simulink model "InitialSystem_9_Bus"  (R2020a)
settings: Solver=FixedStepAuto  StartTime=0.0  StopTime=Tend  MaxStep=5.0E-5  RelTol=1e-3
values from neighbouring files (symbols this model uses):
  B_s46 = b_s46*Cb    (= 9.5071761847e-07)    [Data_CaseStudyI.m]    (also in Data_CaseStudyII.m; Data_InitialSystem.m)
  B_s54 = b_s54*Cb    (= 1.05902722057e-06)    [Data_CaseStudyI.m]    (also in Data_CaseStudyII.m; Data_InitialSystem.m)
  B_s69 = b_s69*Cb    (= 2.15415764185e-06)    [Data_CaseStudyI.m]    (also in Data_CaseStudyII.m; Data_InitialSystem.m)
  B_s75 = b_s75*Cb    (= 1.84126323577e-06)    [Data_CaseStudyI.m]    (also in Data_CaseStudyII.m; Data_InitialSystem.m)
  B_s87 = b_s87*Cb    (= 8.96562817417e-07)    [Data_CaseStudyI.m]    (also in Data_CaseStudyII.m; Data_InitialSystem.m)
  B_s98 = b_s98*Cb    (= 1.25759482443e-06)    [Data_CaseStudyI.m]    (also in Data_CaseStudyII.m; Data_InitialSystem.m)
  fb = 50    [Data_CaseStudyI.m]    (also in Data_CaseStudyII.m; Data_InitialSystem.m)
  HGov_dyn = HGov_delay*H_tr_droop    [Data_CaseStudyI.m]    (also in Data_CaseStudyII.m; Data_InitialSystem.m)
  HTurb_tot = H_water_way    [Data_CaseStudyI.m]    (also in Data_CaseStudyII.m; Data_InitialSystem.m)
  l1_MVHV1 = 0    [Data_CaseStudyI.m]    (also in Data_CaseStudyII.m; Data_InitialSystem.m)
  l1_MVHV2 = 0    [Data_CaseStudyI.m]    (also in Data_CaseStudyII.m; Data_InitialSystem.m)
  l1_MVHV3 = 0    [Data_CaseStudyI.m]    (also in Data_CaseStudyII.m; Data_InitialSystem.m)
  l2_MVHV1 = l_s14    (= 0.0576)    [Data_CaseStudyI.m]    (also in Data_CaseStudyII.m; Data_InitialSystem.m)
  l2_MVHV2 = l_s72    (= 0.0625)    [Data_CaseStudyI.m]    (also in Data_CaseStudyII.m; Data_InitialSystem.m)
  l2_MVHV3 = l_s39    (= 0.0586)    [Data_CaseStudyI.m]    (also in Data_CaseStudyII.m; Data_InitialSystem.m)
  L_s46 = l_s46*Lb    (= 0.154915055408)    [Data_CaseStudyI.m]    (also in Data_CaseStudyII.m; Data_InitialSystem.m)
  L_s54 = l_s54*Lb    (= 0.143128040323)    [Data_CaseStudyI.m]    (also in Data_CaseStudyII.m; Data_InitialSystem.m)
  L_s69 = l_s69*Lb    (= 0.286256080645)    [Data_CaseStudyI.m]    (also in Data_CaseStudyII.m; Data_InitialSystem.m)
  L_s75 = l_s75*Lb    (= 0.271101346964)    [Data_CaseStudyI.m]    (also in Data_CaseStudyII.m; Data_InitialSystem.m)
  L_s87 = l_s87*Lb    (= 0.12123786945)    [Data_CaseStudyI.m]    (also in Data_CaseStudyII.m; Data_InitialSystem.m)
  L_s98 = l_s98*Lb    (= 0.16973301723)    [Data_CaseStudyI.m]    (also in Data_CaseStudyII.m; Data_InitialSystem.m)
  P_L = pL*Sb    (= 300000000)    [Data_CaseStudyI.m]    (also in Data_CaseStudyII.m; Data_InitialSystem.m)
  p_set_bus1 = P_set_bus1/SbSG1    (= 0.731707317073)    [Data_CaseStudyI.m]    (also in Data_CaseStudyII.m; Data_InitialSystem.m)
  p_set_bus2 = P_set_bus2/SbSG2    (= 0.756707317073)    [Data_CaseStudyI.m]    (also in Data_CaseStudyII.m; Data_InitialSystem.m)
  p_set_bus3 = P_set_bus3/SbSG3    (= 0.731707317073)    [Data_CaseStudyI.m]    (also in Data_CaseStudyII.m; Data_InitialSystem.m)
  Q_L = qL*Sb    (= 82500000)    [Data_CaseStudyI.m]    (also in Data_CaseStudyII.m; Data_InitialSystem.m)
  r1_MVHV1 = 1e-6    (= 1e-06)    [Data_CaseStudyI.m]    (also in Data_CaseStudyII.m; Data_InitialSystem.m)
  r1_MVHV2 = 1e-6    (= 1e-06)    [Data_CaseStudyI.m]    (also in Data_CaseStudyII.m; Data_InitialSystem.m)
  r1_MVHV3 = 1e-6    (= 1e-06)    [Data_CaseStudyI.m]    (also in Data_CaseStudyII.m; Data_InitialSystem.m)
  r2_MVHV1 = 1e-6    (= 1e-06)    [Data_CaseStudyI.m]    (also in Data_CaseStudyII.m; Data_InitialSystem.m)
  r2_MVHV2 = 1e-6    (= 1e-06)    [Data_CaseStudyI.m]    (also in Data_CaseStudyII.m; Data_InitialSystem.m)
  r2_MVHV3 = 1e-6    (= 1e-06)    [Data_CaseStudyI.m]    (also in Data_CaseStudyII.m; Data_InitialSystem.m)
  R_s46 = r_s46*Zb    (= 8.993)    [Data_CaseStudyI.m]    (also in Data_CaseStudyII.m; Data_InitialSystem.m)
  R_s54 = r_s54*Zb    (= 5.29)    [Data_CaseStudyI.m]    (also in Data_CaseStudyII.m; Data_InitialSystem.m)
  R_s69 = r_s69*Zb    (= 20.631)    [Data_CaseStudyI.m]    (also in Data_CaseStudyII.m; Data_InitialSystem.m)
  R_s75 = r_s75*Zb    (= 16.928)    [Data_CaseStudyI.m]    (also in Data_CaseStudyII.m; Data_InitialSystem.m)
  R_s87 = r_s87*Zb    (= 4.4965)    [Data_CaseStudyI.m]    (also in Data_CaseStudyII.m; Data_InitialSystem.m)
  R_s98 = r_s98*Zb    (= 6.2951)    [Data_CaseStudyI.m]    (also in Data_CaseStudyII.m; Data_InitialSystem.m)
  Rg = 0.03    [Data_CaseStudyI.m]    (also in Data_CaseStudyII.m; Data_InitialSystem.m)
  Sb = 100*10^6    (= 100000000)    [Data_CaseStudyI.m]    (also in Data_CaseStudyII.m; Data_InitialSystem.m)
  SbSG1 = r_b1*100*10^6    (= 250000000)    [Data_CaseStudyI.m]    (also in Data_CaseStudyII.m; Data_InitialSystem.m)
  SbSG2 = r_b2*100*10^6    (= 96000000)    [Data_CaseStudyI.m]    (also in Data_CaseStudyII.m; Data_InitialSystem.m)
  SbSG3 = r_b3*100*10^6    (= 64000000)    [Data_CaseStudyI.m]    (also in Data_CaseStudyII.m; Data_InitialSystem.m)
  SGov_dyn = tf([1],[Tg 1])    [Data_CaseStudyI.m]    (also in Data_CaseStudyII.m; Data_InitialSystem.m)
  St_MVHV1 = Sb    (= 100000000)    [Data_CaseStudyI.m]    (also in Data_CaseStudyII.m; Data_InitialSystem.m)
  St_MVHV2 = Sb    (= 100000000)    [Data_CaseStudyI.m]    (also in Data_CaseStudyII.m; Data_InitialSystem.m)
  St_MVHV3 = Sb    (= 100000000)    [Data_CaseStudyI.m]    (also in Data_CaseStudyII.m; Data_InitialSystem.m)
  STurb_reheat = STurb_ch*STurb_rh    [Data_CaseStudyI.m]    (also in Data_CaseStudyII.m; Data_InitialSystem.m)
  T_load_b6 = 1010    [Data_CaseStudyI.m]    (also in Data_InitialSystem.m)
  T_s_power = 1e-4    (= 0.0001)    [Data_CaseStudyI.m]    (also in Data_CaseStudyII.m; Data_InitialSystem.m)
  VbHV = 230*10^3    (= 230000)    [Data_CaseStudyI.m]    (also in Data_CaseStudyII.m; Data_InitialSystem.m)
  VbMV1 = 16.5*10^3    (= 16500)    [Data_CaseStudyI.m]    (also in Data_CaseStudyII.m; Data_InitialSystem.m)
  VbMV2 = 18.0*10^3    (= 18000)    [Data_CaseStudyI.m]    (also in Data_CaseStudyII.m; Data_InitialSystem.m)
  VbMV3 = 13.8*10^3    (= 13800)    [Data_CaseStudyI.m]    (also in Data_CaseStudyII.m; Data_InitialSystem.m)
undefined symbols (not defined in the file or in its folder): A, B, C, Continuous, Dd, Efd0, gcbh, Ka, Kf, p2set, SbSM2, sps_rtmsupport, spsST1AModel, Ta, Tb, Tb1, Tc, Tc1, Tf, VA0, VAmax, VAmin, VImax, VImin, VRmax, VRmin
libraries: powerlib x55, cstblocks x6, sps_avr x2, simulink_extras x1, simulink x1
(part 1 of 2)
settings Model: SimulationMode=accelerator  Creator=verena  LastModifiedBy=verenahaberle
settings DataIOCC: ExternalInput=getinputstruct(spec1)  FinalStateName=xFinal_is  InitialState=xInitial_InitialSystem  LoadInitialState=on  SaveFinalState=on  SaveOperatingPoint=on  SaveFormat=Array  ReturnWorkspaceOutputs=off  TimeSaveName=tout_is  OutputSaveName=yout_is  SignalLoggingName=logsout_is  DSMLoggingName=dsmout_is
settings OptimizationCC: BlockReduction=off
settings DebuggingCC: UnconnectedInputMsg=none  UnconnectedOutputMsg=none  UnconnectedLineMsg=none  NonCurrentReleaseOperatingPointMsg=warning

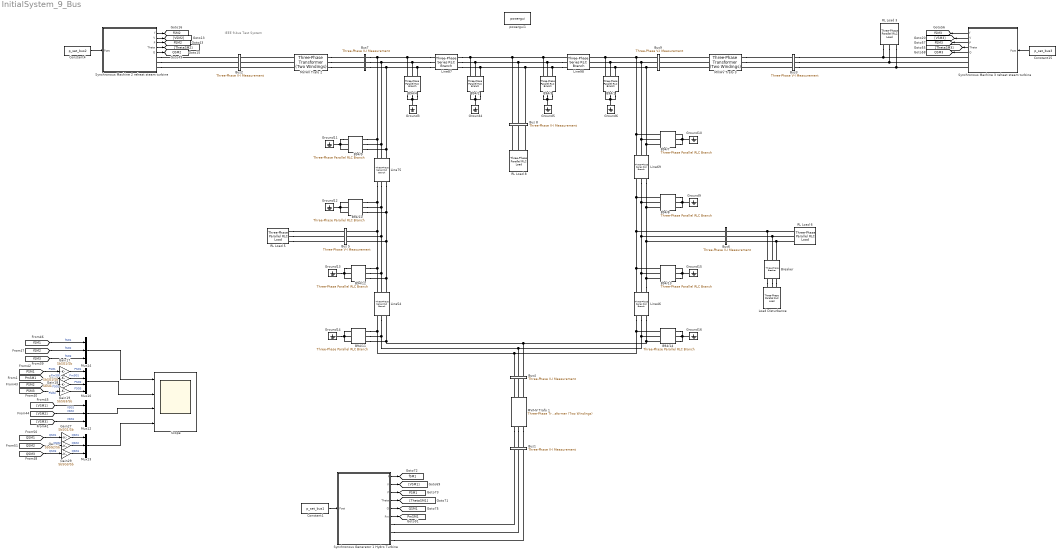
== system InitialSystem_9_Bus ==
  note: IEEE 9-bus Test System
  B94/1 : powerlib/Elements/Three-Phase Parallel RLC Branch  LConnTagsString=A|B|C  RConnTagsString=A|B|C  BranchType=C  Resistance=1  Inductance=1e-3  Capacitance=B_s98*0.5  Measurements=None
      settings: SourceProductBaseCode=PS
  B94/10 : powerlib/Elements/Three-Phase Parallel RLC Branch  LConnTagsString=A|B|C  RConnTagsString=A|B|C  BranchType=C  Resistance=1  Inductance=1e-3  Capacitance=B_s75*0.5  Measurements=None
      settings: SourceProductBaseCode=PS
  B94/11 : powerlib/Elements/Three-Phase Parallel RLC Branch  LConnTagsString=A|B|C  RConnTagsString=A|B|C  BranchType=C  Resistance=1  Inductance=1e-3  Capacitance=B_s54*0.5  Measurements=None
      settings: SourceProductBaseCode=PS
  B94/12 : powerlib/Elements/Three-Phase Parallel RLC Branch  LConnTagsString=A|B|C  RConnTagsString=A|B|C  BranchType=C  Resistance=1  Inductance=1e-3  Capacitance=B_s54*0.5  Measurements=None
      settings: SourceProductBaseCode=PS
  B94/13 : powerlib/Elements/Three-Phase Parallel RLC Branch  LConnTagsString=A|B|C  RConnTagsString=A|B|C  BranchType=C  Resistance=1  Inductance=1e-3  Capacitance=B_s46*0.5  Measurements=None
      settings: SourceProductBaseCode=PS
  B94/14 : powerlib/Elements/Three-Phase Parallel RLC Branch  LConnTagsString=A|B|C  RConnTagsString=A|B|C  BranchType=C  Resistance=1  Inductance=1e-3  Capacitance=B_s46*0.5  Measurements=None
      settings: SourceProductBaseCode=PS
  B94/2 : powerlib/Elements/Three-Phase Parallel RLC Branch  LConnTagsString=A|B|C  RConnTagsString=A|B|C  BranchType=C  Resistance=1  Inductance=1e-3  Capacitance=B_s87*0.5  Measurements=None
      settings: SourceProductBaseCode=PS
  B94/3 : powerlib/Elements/Three-Phase Parallel RLC Branch  LConnTagsString=A|B|C  RConnTagsString=A|B|C  BranchType=C  Resistance=1  Inductance=1e-3  Capacitance=B_s98*0.5  Measurements=None
      settings: SourceProductBaseCode=PS
  B94/4 : powerlib/Elements/Three-Phase Parallel RLC Branch  LConnTagsString=A|B|C  RConnTagsString=A|B|C  BranchType=C  Resistance=1  Inductance=1e-3  Capacitance=B_s87*0.5  Measurements=None
      settings: SourceProductBaseCode=PS
  B94/7 : powerlib/Elements/Three-Phase Parallel RLC Branch  LConnTagsString=A|B|C  RConnTagsString=A|B|C  BranchType=C  Resistance=1  Inductance=1e-3  Capacitance=B_s69*0.5  Measurements=None
      settings: SourceProductBaseCode=PS
  B94/8 : powerlib/Elements/Three-Phase Parallel RLC Branch  LConnTagsString=A|B|C  RConnTagsString=A|B|C  BranchType=C  Resistance=1  Inductance=1e-3  Capacitance=B_s69*0.5  Measurements=None
      settings: SourceProductBaseCode=PS
  B94/9 : powerlib/Elements/Three-Phase Parallel RLC Branch  LConnTagsString=A|B|C  RConnTagsString=A|B|C  BranchType=C  Resistance=1  Inductance=1e-3  Capacitance=B_s75*0.5  Measurements=None
      settings: SourceProductBaseCode=PS
  Breaker : powerlib/Elements/Three-Phase Breaker  InitialState=open  SwitchA=on  SwitchB=on  SwitchC=on  SwitchTimes=[T_load_b6]  External=off  BreakerResistance=0.01  SnubberResistance=1e6  SnubberCapacitance=inf  Measurements=None
  Bus 5 : powerlib/Measurements/Three-Phase V-I Measurement  VoltageMeasurement=no  SetLabelV=on  LabelV=Vabc_5  Vpu=on  VpuLL=off  CurrentMeasurement=no  SetLabelI=on  LabelI=Iabc_5  Ipu=on  Pbase=S_b  Vbase=V_b  OutputType=Complex  PhasorSimulation=off  PSBequivalent=0
  Bus 8 : powerlib/Measurements/Three-Phase V-I Measurement  VoltageMeasurement=no  SetLabelV=on  LabelV=Vabc_9  Vpu=on  VpuLL=off  CurrentMeasurement=no  SetLabelI=on  LabelI=Iabc_9  Ipu=on  Pbase=S_b  Vbase=V_b  OutputType=Complex  PhasorSimulation=off  PSBequivalent=0
  Bus1 : powerlib/Measurements/Three-Phase V-I Measurement  VoltageMeasurement=phase-to-ground  SetLabelV=on  LabelV=Vabc_B1  Vpu=off  VpuLL=on  CurrentMeasurement=yes  SetLabelI=on  LabelI=Iabc_B1  Ipu=off  Pbase=S_b  Vbase=VbMV1  OutputType=Complex  PhasorSimulation=off  PSBequivalent=0
  Bus2 : powerlib/Measurements/Three-Phase V-I Measurement  VoltageMeasurement=no  SetLabelV=on  LabelV=Vabc_2  Vpu=off  VpuLL=off  CurrentMeasurement=no  SetLabelI=on  LabelI=Iabc_2  Ipu=on  Pbase=Sb  Vbase=VbMV2  OutputType=Complex  PhasorSimulation=off  PSBequivalent=0
  Bus3 : powerlib/Measurements/Three-Phase V-I Measurement  VoltageMeasurement=phase-to-ground  SetLabelV=on  LabelV=Vabc_B3  Vpu=off  VpuLL=on  CurrentMeasurement=yes  SetLabelI=on  LabelI=Iabc_B3  Ipu=off  Pbase=S_b  Vbase=VbMV3  OutputType=Complex  PhasorSimulation=off  PSBequivalent=0
  Bus4 : powerlib/Measurements/Three-Phase V-I Measurement  VoltageMeasurement=no  SetLabelV=off  LabelV=Vabc_6  Vpu=off  VpuLL=off  CurrentMeasurement=no  SetLabelI=off  LabelI=Iabc_6  Ipu=off  Pbase=S_b  Vbase=V_b  OutputType=Complex  PhasorSimulation=off  PSBequivalent=0
  Bus6 : powerlib/Measurements/Three-Phase V-I Measurement  VoltageMeasurement=no  SetLabelV=on  LabelV=Vabc_9  Vpu=on  VpuLL=off  CurrentMeasurement=no  SetLabelI=on  LabelI=Iabc_9  Ipu=on  Pbase=S_b  Vbase=V_b  OutputType=Complex  PhasorSimulation=off  PSBequivalent=0
  Bus7 : powerlib/Measurements/Three-Phase V-I Measurement  VoltageMeasurement=no  SetLabelV=on  LabelV=Vabc_4  Vpu=on  VpuLL=off  CurrentMeasurement=no  SetLabelI=on  LabelI=Iabc_4  Ipu=on  Pbase=S_b  Vbase=V_b  OutputType=Complex  PhasorSimulation=off  PSBequivalent=0
  Bus9 : powerlib/Measurements/Three-Phase V-I Measurement  VoltageMeasurement=phase-to-ground  SetLabelV=on  LabelV=Vabc_9  Vpu=off  VpuLL=off  CurrentMeasurement=yes  SetLabelI=on  LabelI=Iabc_9  Ipu=off  Pbase=S_b  Vbase=V_b  OutputType=Complex  PhasorSimulation=off  PSBequivalent=0
  Constant1 : Constant  Value=p_set_bus1
  Constant15 : Constant  Value=p_set_bus3
  Constant4 : Constant  Value=p_set_bus2
  Gain1 : Gain  Gain=SbSG1/Sb
  Gain17 : Gain  Gain=SbSG1/Sb
  Gain18 : Gain  Gain=SbSG2/Sb
  Gain19 : Gain  Gain=SbSG3/Sb
  Gain27 : Gain  Gain=SbSG1/Sb
  Gain28 : Gain  Gain=SbSG2/Sb
  Gain29 : Gain  Gain=SbSG3/Sb
  Ground{3..6,9..16} (12 alike) : powerlib/Elements/Ground  LConnTagsString=a
  Line46 : powerlib/Elements/Three-Phase Series RLC Branch  LConnTagsString=A|B|C  RConnTagsString=A|B|C  BranchType=RL  Resistance=R_s46  Inductance=L_s46  Capacitance=0  Measurements=None
  Line54 : powerlib/Elements/Three-Phase Series RLC Branch  LConnTagsString=A|B|C  RConnTagsString=A|B|C  BranchType=RL  Resistance=R_s54  Inductance=L_s54  Capacitance=0  Measurements=None
  Line69 : powerlib/Elements/Three-Phase Series RLC Branch  LConnTagsString=A|B|C  RConnTagsString=A|B|C  BranchType=RL  Resistance=R_s69  Inductance=L_s69  Capacitance=0  Measurements=None
  Line75 : powerlib/Elements/Three-Phase Series RLC Branch  LConnTagsString=A|B|C  RConnTagsString=A|B|C  BranchType=RL  Resistance=R_s75  Inductance=L_s75  Capacitance=0  Measurements=None
  Line87 : powerlib/Elements/Three-Phase Series RLC Branch  LConnTagsString=A|B|C  RConnTagsString=A|B|C  BranchType=RL  Resistance=R_s87  Inductance=L_s87  Capacitance=0  Measurements=None
  Line98 : powerlib/Elements/Three-Phase Series RLC Branch  LConnTagsString=A|B|C  RConnTagsString=A|B|C  BranchType=RL  Resistance=R_s98  Inductance=L_s98  Capacitance=0  Measurements=None
  Load Disturbance : powerlib/Elements/Three-Phase Parallel RLC Load  LConnTagsString=A|B|C  Configuration=Y (grounded)  NominalVoltage=VbHV  Vabc=[1e3 1e3 1e3]  Vabcp=[1e3 1e3 1e3]  NominalFrequency=fb  UnbalancedPower=off  ActivePower=Load_step_b6  InductivePower=0  CapacitivePower=0  Pabc=[10e3 9e3 11e3]  QLabc=[100 90 110]  QCabc=[100 90 110]  Pabcp=[10e3 9e3 11e3]  QLabcp=[100 90 110]  QCabcp=[100 90 110]  Measurements=None  LoadType=constant Z
  "MV/HV Trafo 1 " : powerlib/Elements/Three-Phase Transformer (Two Windings)  Winding1Connection=Yg  Winding2Connection=Yg  CoreType=Three single-phase transformers  SetSaturation=off  Hysteresis=off  DataFile='hysteresis'  SetInitialFlux=off  Measurements=None  UNITS=pu  NominalPower=[St_MVHV1 fb ]  Winding1=[VbMV1 r1_MVHV1 l1_MVHV1]  Winding2=[VbHV r2_MVHV1 l2_MVHV1]  Rm=500  Lm=500  L0=0.5  Saturation="[ 0,0  ;  0.005,1.2  ;  1.0,1.4 ]"  InitialFluxes=[ 0.8 , -0.8 , 0.7 ]  BreakLoop=off  DiscreteSolver=Backward Euler robust  DataType=off  TransfoNumber=0
  "MV/HV Trafo 2 " : powerlib/Elements/Three-Phase Transformer (Two Windings)  Winding1Connection=Yg  Winding2Connection=Yg  CoreType=Three single-phase transformers  SetSaturation=off  Hysteresis=off  DataFile='hysteresis'  SetInitialFlux=off  Measurements=None  UNITS=pu  NominalPower=[St_MVHV2 fb ]  Winding1=[VbMV2 r1_MVHV2 l1_MVHV2]  Winding2=[ VbHV r2_MVHV2 l2_MVHV2]  Rm=500  Lm=500  L0=0.5  Saturation="[ 0,0  ;  0.005,1.2  ;  1.0,1.4 ]"  InitialFluxes=[ 0.8 , -0.8 , 0.7 ]  BreakLoop=off  DiscreteSolver=Backward Euler robust  DataType=off  TransfoNumber=0
  "MV/HV Trafo 3 " : powerlib/Elements/Three-Phase Transformer (Two Windings)  Winding1Connection=Yg  Winding2Connection=Yg  CoreType=Three single-phase transformers  SetSaturation=off  Hysteresis=off  DataFile='hysteresis'  SetInitialFlux=off  Measurements=None  UNITS=pu  NominalPower=[St_MVHV3 fb ]  Winding1=[VbMV3 r1_MVHV3 l1_MVHV3]  Winding2=[ VbHV r2_MVHV3 l2_MVHV3]  Rm=500  Lm=500  L0=0.5  Saturation="[ 0,0  ;  0.005,1.2  ;  1.0,1.4 ]"  InitialFluxes=[ 0.8 , -0.8 , 0.7 ]  BreakLoop=off  DiscreteSolver=Backward Euler robust  DataType=off  TransfoNumber=0
  Mux10 : Mux
  Mux12 : Mux  Inputs=3
  Mux13 : Mux  Inputs=3
  Mux14 : Mux  Inputs=3
  RL Load 3 : powerlib/Elements/Three-Phase Parallel RLC Load  LConnTagsString=A|B|C  Configuration=Y (grounded)  NominalVoltage=VbMV3  Vabc=[1e3 1e3 1e3]  Vabcp=[1e3 1e3 1e3]  NominalFrequency=fb  UnbalancedPower=off  ActivePower=P_L/12  InductivePower=Q_L/12  CapacitivePower=0  Pabc=[10e3 9e3 11e3]  QLabc=[100 90 110]  QCabc=[100 90 110]  Pabcp=[10e3 9e3 11e3]  QLabcp=[100 90 110]  QCabcp=[100 90 110]  Measurements=None  LoadType=constant Z
  RL Load 5 : powerlib/Elements/Three-Phase Parallel RLC Load  LConnTagsString=A|B|C  Configuration=Y (grounded)  NominalVoltage=VbHV  Vabc=[1e3 1e3 1e3]  Vabcp=[1e3 1e3 1e3]  NominalFrequency=fb  UnbalancedPower=off  ActivePower=P_L/3  InductivePower=Q_L/3  CapacitivePower=0  Pabc=[10e3 9e3 11e3]  QLabc=[100 90 110]  QCabc=[100 90 110]  Pabcp=[10e3 9e3 11e3]  QLabcp=[100 90 110]  QCabcp=[100 90 110]  Measurements=None  LoadType=constant Z
  RL Load 6 : powerlib/Elements/Three-Phase Parallel RLC Load  LConnTagsString=A|B|C  Configuration=Y (grounded)  NominalVoltage=VbHV  Vabc=[1e3 1e3 1e3]  Vabcp=[1e3 1e3 1e3]  NominalFrequency=fb  UnbalancedPower=off  ActivePower=P_L/3  InductivePower=Q_L/3  CapacitivePower=0  Pabc=[10e3 9e3 11e3]  QLabc=[100 90 110]  QCabc=[100 90 110]  Pabcp=[10e3 9e3 11e3]  QLabcp=[100 90 110]  QCabcp=[100 90 110]  Measurements=None  LoadType=constant Z
  "RL Load 8 " : powerlib/Elements/Three-Phase Parallel RLC Load  LConnTagsString=A|B|C  Configuration=Y (grounded)  NominalVoltage=VbHV  Vabc=[1e3 1e3 1e3]  Vabcp=[1e3 1e3 1e3]  NominalFrequency=fb  UnbalancedPower=off  ActivePower=P_L/4  InductivePower=Q_L/4  CapacitivePower=0  Pabc=[10e3 9e3 11e3]  QLabc=[100 90 110]  QCabc=[100 90 110]  Pabcp=[10e3 9e3 11e3]  QLabcp=[100 90 110]  QCabcp=[100 90 110]  Measurements=None  LoadType=constant Z
  Scope : Scope  NumInputPorts=4
  Synchronous Generator 1 Hydro Turbine : Subsystem
  Synchronous Machine 2 reheat steam turbine : Subsystem
  Synchronous Machine 3 reheat steam turbine : Subsystem
  powergui1 : powerlib/powergui  Priority=1  SimulationMode=Discrete  SampleTime=T_s_power  frequency=fb  Iterations=100  frequencyindice=0  Pbase=100e6  ErrMax=0.0001  UnitsV=kV  UnitsW=MW  buscounter=3  FunctionMessages=off  echomessages=off  EnableUseOfTLC=off  CurrentSourceSwitches=off  DisableSnubberDevices=off  DisableRonSwitches=off  DisableVfSwitches=off  DisplayEquations=off  AutomaticDiscreteSolvers=off  SolverType=Tustin/Backward Euler (TBE)  Interpol=off  ExternalGateDelay=off  methode=off  Ts=100  x0status=blocks  SPID=off  SwTol=0  HookPort=off  NonlinearTolerance=1e-5  nMaxIteration=200  ContinueOnMaxIteration=off  RestoreLinks=warning  ResistiveCurrentMeasurement=off  Frange=[0:2:500]  Ylog=off  Xlog=on  ShowGrid=off  save=off  variable=ZData  structure=0  ZoomFFT=off  StartTime=0.0  cycles=1  DisplayStyle=1  fundamental=60  FreqAxis=off  MaxFrequency=1000  frequencyindicesteady=1  RmsSteady=1  display=off
  tag scope: PSM1=global, PSM2=global, PSM3=global, PmSM1=global, QSM1=global, QSM2=global, QSM3=global, fSM1=global, fSM2=global, fSM3=global
  wires:
  Constant4/1 -> Synchronous Machine 2 reheat steam turbine/1(Pset)
  Synchronous Machine 2 reheat steam turbine/1(f) -> [fSM2]
  Synchronous Machine 2 reheat steam turbine/2(V) -> [VSM2]
  Synchronous Machine 2 reheat steam turbine/3(P) -> [PSM2]
  Synchronous Machine 2 reheat steam turbine/4(Theta) -> [ThetaSM2]
  Synchronous Machine 2 reheat steam turbine/5(Q) -> [QSM2]
  Synchronous Machine 3 reheat steam turbine/4(Theta) -> [ThetaSM3]
  Synchronous Machine 3 reheat steam turbine/2(V) -> [VSM3]
  Synchronous Machine 3 reheat steam turbine/3(P) -> [PSM3]
  Constant15/1 -> Synchronous Machine 3 reheat steam turbine/1(Pset)
  Synchronous Machine 3 reheat steam turbine/1(f) -> [fSM3]
  Synchronous Machine 3 reheat steam turbine/5(Q) -> [QSM3]
  Synchronous Generator 1 Hydro Turbine/2(V) -> [VSM1]
  Constant1/1 -> Synchronous Generator 1 Hydro Turbine/1(Pset)
  Synchronous Generator 1 Hydro Turbine/6(Pm) -> [PmSM1]
  Synchronous Generator 1 Hydro Turbine/4(Theta) -> [ThetaSM1]
  Synchronous Generator 1 Hydro Turbine/3(P) -> [PSM1]
  Synchronous Generator 1 Hydro Turbine/5(Q) -> [QSM1]
  Synchronous Generator 1 Hydro Turbine/1(f) -> [fSM1]
  [VSM1] -> Mux12/1  "VSG1"
  [fSM3] -> Mux14/3  "fSG3"
  [PSM2] -> Gain18/1  "PSG2"
  [QSM1] -> Gain27/1  "QSG1"
  Mux14/1 -> Scope/1
  Gain28/1 -> Mux13/2  "QSG2"
  [VSM2] -> Mux12/2  "VSG2"
  [QSM2] -> Gain28/1  "QSG2"
  [PSM3] -> Gain19/1  "PSG3"
  Mux13/1 -> Scope/4
  Mux12/1 -> Scope/3
  Gain27/1 -> Mux13/1  "QSG1"
  [QSM3] -> Gain29/1  "QSG3"
  Gain17/1 -> Mux10/1  "PSG1"
  Gain29/1 -> Mux13/3  "QSG3"
  [fSM2] -> Mux14/2  "fSG2"
  [PSM1] -> Gain17/1  "PSG1"
  [fSM1] -> Mux14/1  "fSG1"
  Mux10/1 -> Scope/2
  [VSM3] -> Mux12/3  "VSG3"
  Gain19/1 -> Mux10/4  "PSG3"
  Gain18/1 -> Mux10/3  "PSG2"
  [PmSM1] -> Gain1/1  "PmSG1"
  Gain1/1 -> Mux10/2  "PmSG1"
  connections:
  B94/1/RConn1 -- Ground6/LConn1 -- B94/1/RConn2 -- B94/1/RConn3
  B94/9/RConn1 -- Ground11/LConn1 -- B94/9/RConn3 -- B94/9/RConn2
  RL Load 6/LConn3 -- Breaker/RConn3 -- Bus6/LConn3
  Bus 5/LConn1 -- Line54/LConn1 -- B94/12/LConn1 -- Line75/RConn1 -- B94/10/LConn1
  "MV/HV Trafo 2 "/RConn1 -- Bus7/RConn1
  "MV/HV Trafo 1 "/LConn1 -- Bus1/LConn1
  B94/3/RConn3 -- B94/3/RConn1 -- B94/3/RConn2 -- Ground5/LConn1
  B94/10/LConn3 -- Line75/RConn3 -- Line54/LConn3 -- B94/12/LConn3 -- Bus 5/LConn3
  B94/13/LConn1 -- Line46/LConn1 -- Bus6/RConn1 -- B94/8/LConn1 -- Line69/RConn1
  B94/8/LConn2 -- B94/13/LConn2 -- Line46/LConn2 -- Bus6/RConn2 -- Line69/RConn2
  Ground16/LConn1 -- B94/14/RConn3 -- B94/14/RConn1 -- B94/14/RConn2
  B94/11/RConn2 -- Ground14/LConn1 -- B94/11/RConn3 -- B94/11/RConn1
  Line87/LConn2 -- B94/4/LConn2 -- Bus7/LConn2 -- Line75/LConn2 -- B94/9/LConn2
  B94/2/RConn1 -- Ground4/LConn1 -- B94/2/RConn2 -- B94/2/RConn3
  "MV/HV Trafo 3 "/LConn1 -- Bus3/LConn1
  Line98/LConn2 -- B94/3/LConn2 -- Bus 8/RConn2 -- B94/2/LConn2 -- Line87/RConn2
  Line98/RConn2 -- B94/1/LConn2 -- B94/7/LConn2 -- Line69/LConn2 -- Bus9/RConn2
  Line98/LConn3 -- B94/3/LConn3 -- Bus 8/RConn1 -- Line87/RConn3 -- B94/2/LConn3
  RL Load 6/LConn1 -- Breaker/RConn1 -- Bus6/LConn1
  B94/11/LConn2 -- Line54/RConn2 -- Line46/RConn2 -- B94/14/LConn2 -- Bus4/LConn2
  Ground12/LConn1 -- B94/10/RConn3 -- B94/10/RConn1 -- B94/10/RConn2
  B94/14/LConn3 -- Line46/RConn3 -- Bus4/LConn3 -- B94/11/LConn3 -- Line54/RConn3
  Line54/RConn1 -- B94/11/LConn1 -- Bus4/LConn1 -- Line46/RConn1 -- B94/14/LConn1
  "MV/HV Trafo 3 "/RConn1 -- Bus9/LConn1
  B94/2/LConn1 -- Line87/RConn1 -- Bus 8/RConn3 -- B94/3/LConn1 -- Line98/LConn1
  Line98/RConn3 -- B94/1/LConn3 -- Bus9/RConn3 -- B94/7/LConn3 -- Line69/LConn3
  Line87/LConn3 -- B94/4/LConn3 -- Bus7/LConn3 -- B94/9/LConn3 -- Line75/LConn3
  Line46/LConn3 -- B94/8/LConn3 -- Line69/RConn3 -- Bus6/RConn3 -- B94/13/LConn3
  "MV/HV Trafo 2 "/LConn1 -- Bus2/LConn1
  B94/8/RConn3 -- B94/8/RConn1 -- B94/8/RConn2 -- Ground9/LConn1
  Line98/RConn1 -- B94/1/LConn1 -- Bus9/RConn1 -- B94/7/LConn1 -- Line69/LConn1
  B94/10/LConn2 -- Line75/RConn2 -- Line54/LConn2 -- B94/12/LConn2 -- Bus 5/LConn2
  B94/4/RConn3 -- B94/4/RConn1 -- B94/4/RConn2 -- Ground3/LConn1
  Line87/LConn1 -- B94/4/LConn1 -- B94/9/LConn1 -- Line75/LConn1 -- Bus7/LConn1
  B94/7/RConn1 -- Ground10/LConn1 -- B94/7/RConn3 -- B94/7/RConn2
  B94/12/RConn1 -- Ground13/LConn1 -- B94/12/RConn3 -- B94/12/RConn2
  RL Load 6/LConn2 -- Breaker/RConn2 -- Bus6/LConn2
  B94/13/RConn1 -- Ground15/LConn1 -- B94/13/RConn3 -- B94/13/RConn2
  Synchronous Machine 2 reheat steam turbine/RConn3 -- Bus2/RConn3
  "RL Load 8 "/LConn3 -- Bus 8/LConn1
  "MV/HV Trafo 3 "/LConn2 -- Bus3/LConn2
  "MV/HV Trafo 3 "/RConn2 -- Bus9/LConn2
  "MV/HV Trafo 1 "/LConn3 -- Bus1/LConn3
  "MV/HV Trafo 1 "/RConn1 -- Bus4/RConn1
  "MV/HV Trafo 2 "/RConn3 -- Bus7/RConn3
  RL Load 5/LConn2 -- Bus 5/RConn2
  "MV/HV Trafo 2 "/RConn2 -- Bus7/RConn2
  "MV/HV Trafo 1 "/RConn2 -- Bus4/RConn2
  "RL Load 8 "/LConn2 -- Bus 8/LConn2
  "MV/HV Trafo 2 "/LConn2 -- Bus2/LConn2
  RL Load 5/LConn3 -- Bus 5/RConn3
  "RL Load 8 "/LConn1 -- Bus 8/LConn3
  Synchronous Machine 2 reheat steam turbine/RConn1 -- Bus2/RConn1
  "MV/HV Trafo 2 "/LConn3 -- Bus2/LConn3
  "MV/HV Trafo 1 "/LConn2 -- Bus1/LConn2
  "MV/HV Trafo 3 "/RConn3 -- Bus9/LConn3
  RL Load 5/LConn1 -- Bus 5/RConn1
  Synchronous Machine 2 reheat steam turbine/RConn2 -- Bus2/RConn2
  "MV/HV Trafo 1 "/RConn3 -- Bus4/RConn3
  Bus3/LConn3 -- "MV/HV Trafo 3 "/LConn3
  RL Load 3/LConn3 -- Synchronous Machine 3 reheat steam turbine/RConn3 -- Bus3/RConn3
  Synchronous Generator 1 Hydro Turbine/RConn2 -- Bus1/RConn2
  Synchronous Generator 1 Hydro Turbine/RConn3 -- Bus1/RConn3
  Synchronous Generator 1 Hydro Turbine/RConn1 -- Bus1/RConn1
  Breaker/LConn3 -- Load Disturbance/LConn3
  Breaker/LConn1 -- Load Disturbance/LConn1
  Breaker/LConn2 -- Load Disturbance/LConn2
  RL Load 3/LConn2 -- Synchronous Machine 3 reheat steam turbine/RConn2 -- Bus3/RConn2
  Bus3/RConn1 -- RL Load 3/LConn1 -- Synchronous Machine 3 reheat steam turbine/RConn1

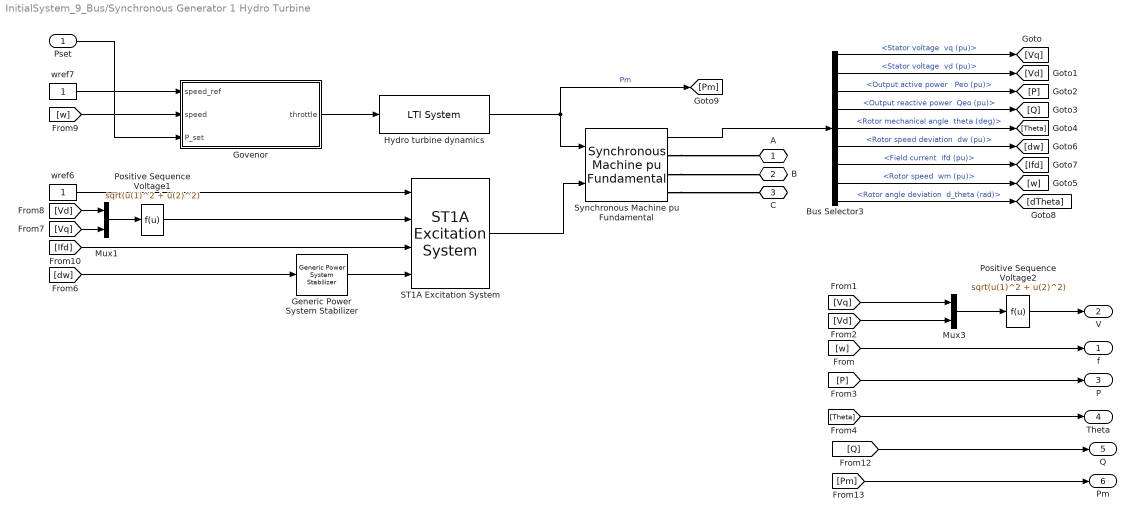
== system InitialSystem_9_Bus/Synchronous Generator 1 Hydro Turbine ==
  Pset : Inport
  Bus Selector3 : BusSelector  OutputSignals="dq0 components.Stator voltage  vq (pu),dq0 components.Stator voltage  vd (pu),Output active power   Peo (pu),Output reactive power  Qeo (pu),Mechanical.Rotor mechanical angle  theta (deg),Mechanical.Rotor speed deviation  dw (pu),dq0 components.Field current  ifd (pu),Mechanical.Rotor speed  wm (pu),Mechanical.Rotor angle deviation  d_theta (rad)"
  Generic Power System Stabilizer : powerlib/Machines/Generic Power System Stabilizer  Tsensor=30e-3  K=15  Twashout=1  Tleadlag1=[50e-3 20e-3]  Tleadlag2=[3 5.4]  VSlimits=[-0.15 0.15]  Vinit=0  Plot_On=off  MagdB_On=on  FreqRange=logspace(-2,2,500)
      settings: SourceProductBaseCode=PS
  Govenor : Subsystem
  Hydro turbine dynamics : cstblocks/LTI System  sys=ss(HTurb_tot)  IC=p_set_bus1/3
  Mux1 : Mux  Inputs=2
  Mux3 : Mux  Inputs=2
  Positive Sequence Voltage1 : Fcn  Expr=sqrt(u(1)^2 + u(2)^2)
  Positive Sequence Voltage2 : Fcn  Expr=sqrt(u(1)^2 + u(2)^2)
  ST1A Excitation System : sps_avr/ST1A Excitation System  Tr=20e-3  KaTa=[210 0.001]  VIminmax=[-999 +999]  VAminmax=[-999 999]  VRminmax=[-6.0 6.43]  KfTf=[0.001 1]  TbTc=[0 0 0 0]  KLR=1  ILR=2  Kc=0.038  v0=[1 1.7165]  TsBlock=0
      settings: SourceProductBaseCode=PS
  Synchronous Machine pu Fundamental : powerlib/Machines/Synchronous Machine pu Fundamental  PresetModel=No  MechanicalLoad=Mechanical power Pm  ShowDetailedParameters=on  RotorType=Round  Units=per unit fundamental parameters  MeasurementBus=off  NominalParameters="[SbSG1  VbMV1   fb]"  Stator="[ 2.85E-03  0.114  1.19  0.36 ]"  Field="[ 5.79E-04  0.114]"  Dampers2=[0.0652, 0.5134, 0.0287, 0.2553, 7.765e-3, 0.9167 ]  Dampers1="[ 1.17E-02  0.182  1.97E-02  0.384 ]"  Mechanical=[6 0.0032 20]  PolePairs=20  InitialConditions=[0 0 0 0 0 0 0 0 1]  SetSaturation=off  Saturation=[0.6404,0.7127,0.8441,0.9214,0.9956,1.082,1.19,1.316,1.457;0.7,0.7698,0.8872,0.9466,0.9969,1.046,1.1,1.151,1.201]  LoadFlowParameters=[1,0,0,0,0]  TsPowergui=0  TsBlock=-1  IterativeModel=Trapezoidal non iterative  IterativeDiscreteModel=Trapezoidal non iterative  BusType=swing  Pref=p2set*SbSM2  Qref=0  Qmin=-inf  Qmax=inf  PLF=0  QLF=0
      settings: SourceProductBaseCode=PS
  wref6 : Constant
  wref7 : Constant
  A : PMIOPort  Side=Right
  B : PMIOPort  Port=2  Side=Right
  C : PMIOPort  Port=3  Side=Right
  f : Outport  VectorParamsAs1DForOutWhenUnconnected=off
  V : Outport  Port=2  VectorParamsAs1DForOutWhenUnconnected=off
  P : Outport  Port=3  VectorParamsAs1DForOutWhenUnconnected=off
  Theta : Outport  Port=4  VectorParamsAs1DForOutWhenUnconnected=off
  Q : Outport  Port=5  VectorParamsAs1DForOutWhenUnconnected=off
  Pm : Outport  Port=6  VectorParamsAs1DForOutWhenUnconnected=off
  wires:
  ST1A Excitation System/1 -> Synchronous Machine pu Fundamental/2
  [dw] -> Generic Power System Stabilizer/1
  Bus Selector3/8 -> [w]  "<Rotor speed  wm (pu)>"
  Bus Selector3/7 -> [Ifd]  "<Field current  ifd (pu)>"
  Bus Selector3/6 -> [dw]  "<Rotor speed deviation  dw (pu)>"
  Bus Selector3/5 -> [Theta]  "<Rotor mechanical angle  theta (deg)>"
  Bus Selector3/4 -> [Q]  "<Output reactive power  Qeo (pu)>"
  Bus Selector3/3 -> [P]  "<Output active power   Peo (pu)>"
  Bus Selector3/2 -> [Vd]  "<Stator voltage  vd (pu)>"
  Bus Selector3/1 -> [Vq]  "<Stator voltage  vq (pu)>"
  [Theta] -> Theta/1
  [P] -> P/1
  [Vd] -> Mux3/2
  [Vq] -> Mux3/1
  Synchronous Machine pu Fundamental/1 -> Bus Selector3/1
  Mux3/1 -> Positive Sequence Voltage2/1
  wref6/1 -> ST1A Excitation System/1
  Positive Sequence Voltage2/1 -> V/1
  [w] -> f/1
  Bus Selector3/9 -> [dTheta]  "<Rotor angle deviation  d_theta (rad)>"
  Mux1/1 -> Positive Sequence Voltage1/1
  [Vd] -> Mux1/1
  [Vq] -> Mux1/2
  Generic Power System Stabilizer/1 -> ST1A Excitation System/4
  Govenor/1(throttle) -> Hydro turbine dynamics/1
  [Q] -> Q/1
  Positive Sequence Voltage1/1 -> ST1A Excitation System/2
  [Ifd] -> ST1A Excitation System/3
  wref7/1 -> Govenor/1(speed_ref)
  Pset/1 -> Govenor/3(P_set)
  [Pm] -> Pm/1
  [w] -> Govenor/2(speed)
  Hydro turbine dynamics/1 -> Synchronous Machine pu Fundamental/1, [Pm]  "Pm"
  connections:
  Synchronous Machine pu Fundamental/RConn2 -- B/RConn1
  Synchronous Machine pu Fundamental/RConn3 -- C/RConn1
  Synchronous Machine pu Fundamental/RConn1 -- A/RConn1

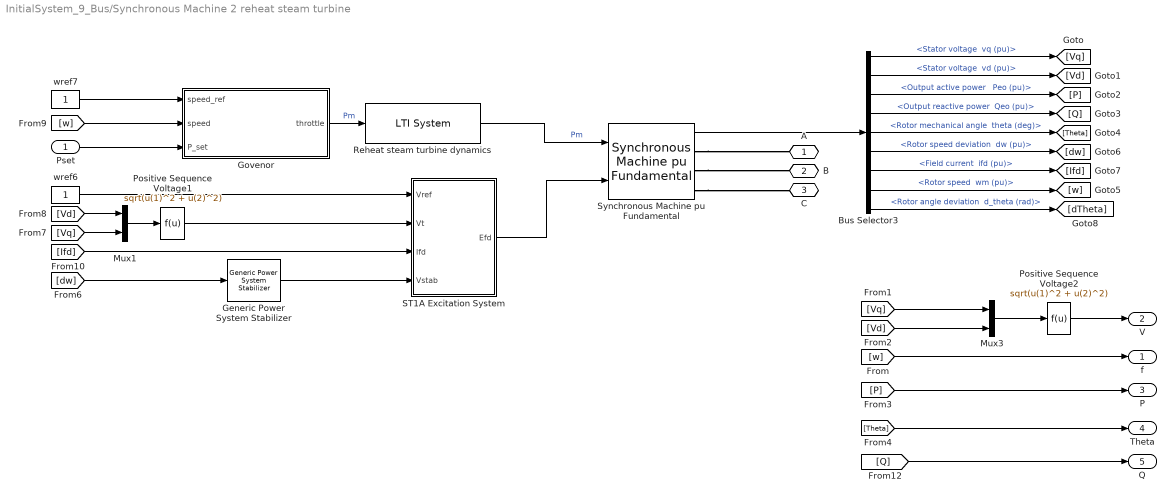
== system InitialSystem_9_Bus/Synchronous Machine 2 reheat steam turbine ==
  Pset : Inport
  Bus Selector3 : BusSelector  OutputSignals="dq0 components.Stator voltage  vq (pu),dq0 components.Stator voltage  vd (pu),Output active power   Peo (pu),Output reactive power  Qeo (pu),Mechanical.Rotor mechanical angle  theta (deg),Mechanical.Rotor speed deviation  dw (pu),dq0 components.Field current  ifd (pu),Mechanical.Rotor speed  wm (pu),Mechanical.Rotor angle deviation  d_theta (rad)"
  Generic Power System Stabilizer : powerlib/Machines/Generic Power System Stabilizer  Tsensor=30e-3  K=15  Twashout=1  Tleadlag1=[50e-3 20e-3]  Tleadlag2=[3 5.4]  VSlimits=[-0.15 0.15]  Vinit=0  Plot_On=off  MagdB_On=on  FreqRange=logspace(-2,2,500)
      settings: SourceProductBaseCode=PS
  Govenor : Subsystem
  Mux1 : Mux  Inputs=2
  Mux3 : Mux  Inputs=2
  Positive Sequence Voltage1 : Fcn  Expr=sqrt(u(1)^2 + u(2)^2)
  Positive Sequence Voltage2 : Fcn  Expr=sqrt(u(1)^2 + u(2)^2)
  Reheat steam turbine dynamics : cstblocks/LTI System  sys=ss(STurb_reheat)  IC=[1 0.2281]
  ST1A Excitation System : Subsystem  AncestorBlock=sps_avr/ST1A Excitation System  DialogController=POWERSYS.PowerSysDialog  LoadFcn=sps_rtmsupport('LoadFcn', gcbh);  StartFcn=sps_rtmsupport('StartFcn', gcbh);  StopFcn=sps_rtmsupport('StopFcn', gcbh);  mask(ST1A Excitation System){Tr=20e-3, KaTa=[210 0.001], VIminmax=[-999 +999], VAminmax=[-999 999], VRminmax=[-6.0 6.43], KfTf=[0.001 1], TbTc=[0 0 0 0], KLR=1, ILR=2, Kc=0.038, v0=[1 1.6825], TsBlock=0}
      mask prompts: Tr "Low-pass filter time constant Tr(s):"; KaTa "Voltage regulator gain and time constant [Ka Ta(s)]:"; VIminmax "Voltage regulator input limits [VImin(pu) VImax(pu)]:"; VAminmax "Voltage regulator internal limits [VAmin(pu) VAmax(pu)]:"; VRminmax "Voltage regulator output limits [VRmin(pu) VRmax(pu)]:"; KfTf "Damping filter gain and time constant [Kf Tf(s)]:"; TbTc "Transient gain reduction lead and lag time constants [Tb(s) Tc(s) Tb1(s) Tc1(s)]:"; KLR "Exciter output current limiter gain KLR(pu):"; ILR "Exciter output current limit reference ILR(pu):"; Kc "Rectifier loading factor Kc(pu):"; v0 "Initial values of terminal voltage and field voltage [Vt0(pu) Efd0(pu)]:"; TsBlock "Sample time:"
      mask help: Implements a synchronous machine voltage regulator and exciter based on the IEEE type ST1A excitation system model. The output is the field voltage to apply to the Vf input of a Synchronous Machine block. Inputs and output are in p.u.
      mask init:
      | block = gcb;
      | [Ts,BlockChoice,MaskType,Ka,Ta,Kf,Tf,Tb,Tc,Tb1,Tc1,VRmin,VRmax,VImin,VImax,VAmin,VAmax,Ifd0,VA0,Vt0,Efd0] = powericon('ExcitationSystemInit',block,TsBlock,KaTa,KfTf,TbTc,VRminmax,VIminmax,VAminmax,Kc,ILR,KLR,v0);
      | powericon('SetInternalModels','set',block,BlockChoice);
      settings: CopyFcn=sps_rtmsupport('CopyFcn', gcbh);  DeleteFcn=sps_rtmsupport('DeleteFcn', gcbh);  UndoDeleteFcn=sps_rtmsupport('UndoDeleteFcn', gcbh);  ModelCloseFcn=sps_rtmsupport('ModelCloseFcn', gcbh);  PreSaveFcn=sps_rtmsupport('PreSaveFcn', gcbh);  PostSaveFcn=sps_rtmsupport('PostSaveFcn', gcbh);  NameChangeFcn=sps_rtmsupport('NameChangeFcn', gcbh);  PreCopyFcn=sps_rtmsupport('PreCopyFcn', gcbh);  OpenFcn=sps_rtmsupport('OpenFcn', gcbh, []);  CloseFcn=sps_rtmsupport('CloseFcn', gcbh);  PreDeleteFcn=sps_rtmsupport('PreDeleteFcn', gcbh);
      mask Help: helpview(psbhelp);
      mask Display: color('blue');disp('ST1A')
  Synchronous Machine pu Fundamental : powerlib/Machines/Synchronous Machine pu Fundamental  PresetModel=No  MechanicalLoad=Mechanical power Pm  ShowDetailedParameters=on  RotorType=Round  Units=per unit fundamental parameters  MeasurementBus=off  NominalParameters="[ SbSG2  VbMV2   fb]"  Stator="[ 2.85E-03  0.114  1.19  0.36 ]"  Field="[ 5.79E-04  0.114]"  Dampers2=[0.0652, 0.5134, 0.0287, 0.2553, 7.765e-3, 0.9167 ]  Dampers1="[ 1.17E-02  0.182  1.97E-02  0.384 ]"  Mechanical=[13 0 20]  PolePairs=20  InitialConditions=[0 0 0 0 0 0 0 0 1]  SetSaturation=off  Saturation=[0.6404,0.7127,0.8441,0.9214,0.9956,1.082,1.19,1.316,1.457;0.7,0.7698,0.8872,0.9466,0.9969,1.046,1.1,1.151,1.201]  LoadFlowParameters=[1,0,0,0,0]  TsPowergui=0  TsBlock=-1  IterativeModel=Trapezoidal non iterative  IterativeDiscreteModel=Trapezoidal non iterative  BusType=PV  Pref=P_set_bus2  Qref=0  Qmin=-inf  Qmax=inf  PLF=0  QLF=0
      settings: SourceProductBaseCode=PS
  wref6 : Constant
  wref7 : Constant
  A : PMIOPort  Side=Right
  B : PMIOPort  Port=2  Side=Right
  C : PMIOPort  Port=3  Side=Right
  f : Outport  VectorParamsAs1DForOutWhenUnconnected=off
  V : Outport  Port=2  VectorParamsAs1DForOutWhenUnconnected=off
  P : Outport  Port=3  VectorParamsAs1DForOutWhenUnconnected=off
  Theta : Outport  Port=4  VectorParamsAs1DForOutWhenUnconnected=off
  Q : Outport  Port=5  VectorParamsAs1DForOutWhenUnconnected=off
  wires:
  ST1A Excitation System/1(Efd) -> Synchronous Machine pu Fundamental/2
  [dw] -> Generic Power System Stabilizer/1
  Generic Power System Stabilizer/1 -> ST1A Excitation System/4(Vstab)
  Bus Selector3/8 -> [w]  "<Rotor speed  wm (pu)>"
  Bus Selector3/7 -> [Ifd]  "<Field current  ifd (pu)>"
  Bus Selector3/6 -> [dw]  "<Rotor speed deviation  dw (pu)>"
  Bus Selector3/5 -> [Theta]  "<Rotor mechanical angle  theta (deg)>"
  Bus Selector3/4 -> [Q]  "<Output reactive power  Qeo (pu)>"
  Bus Selector3/3 -> [P]  "<Output active power   Peo (pu)>"
  Bus Selector3/2 -> [Vd]  "<Stator voltage  vd (pu)>"
  Bus Selector3/1 -> [Vq]  "<Stator voltage  vq (pu)>"
  [Theta] -> Theta/1
  [P] -> P/1
  [Vd] -> Mux3/2
  [Vq] -> Mux3/1
  Synchronous Machine pu Fundamental/1 -> Bus Selector3/1
  Mux3/1 -> Positive Sequence Voltage2/1
  wref6/1 -> ST1A Excitation System/1(Vref)
  Positive Sequence Voltage2/1 -> V/1
  [w] -> f/1
  Bus Selector3/9 -> [dTheta]  "<Rotor angle deviation  d_theta (rad)>"
  Mux1/1 -> Positive Sequence Voltage1/1
  [Vd] -> Mux1/1
  [Vq] -> Mux1/2
  [w] -> Govenor/2(speed)
  wref7/1 -> Govenor/1(speed_ref)
  [Q] -> Q/1
  Govenor/1(throttle) -> Reheat steam turbine dynamics/1  "Pm"
  Positive Sequence Voltage1/1 -> ST1A Excitation System/2(Vt)
  [Ifd] -> ST1A Excitation System/3(Ifd)
  Pset/1 -> Govenor/3(P_set)
  Reheat steam turbine dynamics/1 -> Synchronous Machine pu Fundamental/1  "Pm"
  connections:
  Synchronous Machine pu Fundamental/RConn2 -- B/RConn1
  Synchronous Machine pu Fundamental/RConn3 -- C/RConn1
  Synchronous Machine pu Fundamental/RConn1 -- A/RConn1

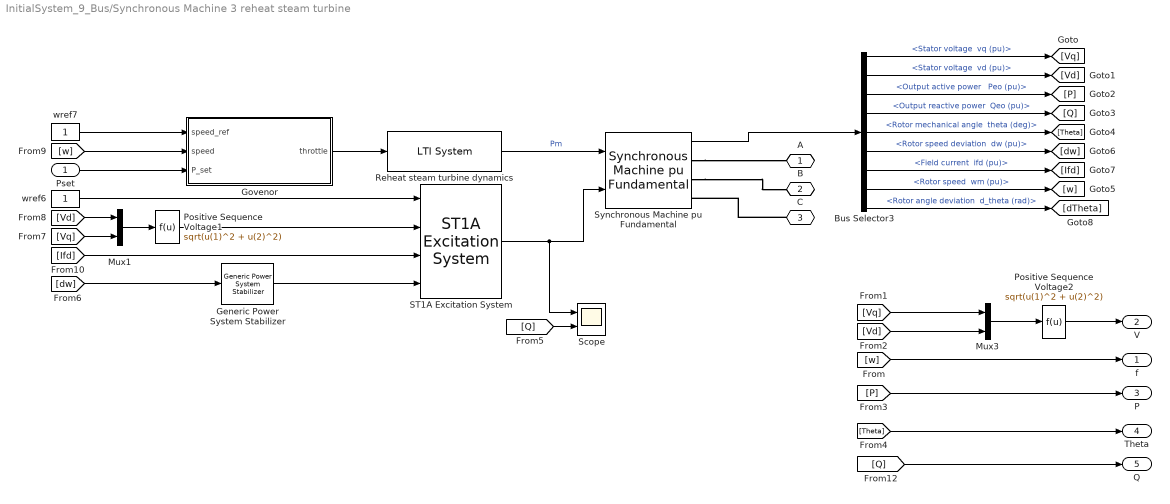
== system InitialSystem_9_Bus/Synchronous Machine 3 reheat steam turbine ==
  Pset : Inport
  Bus Selector3 : BusSelector  OutputSignals="dq0 components.Stator voltage  vq (pu),dq0 components.Stator voltage  vd (pu),Output active power   Peo (pu),Output reactive power  Qeo (pu),Mechanical.Rotor mechanical angle  theta (deg),Mechanical.Rotor speed deviation  dw (pu),dq0 components.Field current  ifd (pu),Mechanical.Rotor speed  wm (pu),Mechanical.Rotor angle deviation  d_theta (rad)"
  Generic Power System Stabilizer : powerlib/Machines/Generic Power System Stabilizer  Tsensor=30e-3  K=15  Twashout=1  Tleadlag1=[50e-3 20e-3]  Tleadlag2=[3 5.4]  VSlimits=[-0.15 0.15]  Vinit=0  Plot_On=off  MagdB_On=on  FreqRange=logspace(-2,2,500)
      settings: SourceProductBaseCode=PS
  Govenor : Subsystem
  Mux1 : Mux  Inputs=2
  Mux3 : Mux  Inputs=2
  Positive Sequence Voltage1 : Fcn  Expr=sqrt(u(1)^2 + u(2)^2)
  Positive Sequence Voltage2 : Fcn  Expr=sqrt(u(1)^2 + u(2)^2)
  Reheat steam turbine dynamics : cstblocks/LTI System  sys=ss(STurb_reheat)  IC=[1 0.2281]
  ST1A Excitation System : sps_avr/ST1A Excitation System  Tr=20e-3  KaTa=[210 0.001]  VIminmax=[-999 +999]  VAminmax=[-999 999]  VRminmax=[-6.0 6.43]  KfTf=[0.001 1]  TbTc=[0 0 0 0]  KLR=1  ILR=2  Kc=0.038  v0=[1 1.64]  TsBlock=0
      settings: SourceProductBaseCode=PS
  Scope : Scope  NumInputPorts=2
  Synchronous Machine pu Fundamental : powerlib/Machines/Synchronous Machine pu Fundamental  PresetModel=No  MechanicalLoad=Mechanical power Pm  ShowDetailedParameters=on  RotorType=Round  Units=per unit fundamental parameters  MeasurementBus=off  NominalParameters="[ SbSG3 VbMV3   fb]"  Stator="[ 2.85E-03  0.114  1.19  0.36 ]"  Field="[ 5.79E-04  0.114]"  Dampers2=[0.0652, 0.5134, 0.0287, 0.2553, 7.765e-3, 0.9167 ]  Dampers1="[ 1.17E-02  0.182  1.97E-02  0.384 ]"  Mechanical=[13 0 20]  PolePairs=20  InitialConditions=[0 -61.0946 1.01786 1.01786 1.01786 6.04511 -113.955 126.045 1.41461]  SetSaturation=off  Saturation=[0.6404,0.7127,0.8441,0.9214,0.9956,1.082,1.19,1.316,1.457;0.7,0.7698,0.8872,0.9466,0.9969,1.046,1.1,1.151,1.201]  LoadFlowParameters=[1,0,0,0,0]  TsPowergui=0  TsBlock=-1  IterativeModel=Trapezoidal non iterative  IterativeDiscreteModel=Trapezoidal non iterative  BusType=PV  Pref=P_set_bus3  Qref=0  Qmin=-inf  Qmax=inf  PLF=0  QLF=0
      settings: SourceProductBaseCode=PS
  wref6 : Constant
  wref7 : Constant
  A : PMIOPort  Side=Right
  B : PMIOPort  Port=2  Side=Right
  C : PMIOPort  Port=3  Side=Right
  f : Outport  VectorParamsAs1DForOutWhenUnconnected=off
  V : Outport  Port=2  VectorParamsAs1DForOutWhenUnconnected=off
  P : Outport  Port=3  VectorParamsAs1DForOutWhenUnconnected=off
  Theta : Outport  Port=4  VectorParamsAs1DForOutWhenUnconnected=off
  Q : Outport  Port=5  VectorParamsAs1DForOutWhenUnconnected=off
  wires:
  ST1A Excitation System/1 -> Scope/1, Synchronous Machine pu Fundamental/2
  [dw] -> Generic Power System Stabilizer/1
  Generic Power System Stabilizer/1 -> ST1A Excitation System/4
  Bus Selector3/8 -> [w]  "<Rotor speed  wm (pu)>"
  Bus Selector3/7 -> [Ifd]  "<Field current  ifd (pu)>"
  Bus Selector3/6 -> [dw]  "<Rotor speed deviation  dw (pu)>"
  Bus Selector3/5 -> [Theta]  "<Rotor mechanical angle  theta (deg)>"
  Bus Selector3/4 -> [Q]  "<Output reactive power  Qeo (pu)>"
  Bus Selector3/3 -> [P]  "<Output active power   Peo (pu)>"
  Bus Selector3/2 -> [Vd]  "<Stator voltage  vd (pu)>"
  Bus Selector3/1 -> [Vq]  "<Stator voltage  vq (pu)>"
  [Theta] -> Theta/1
  [P] -> P/1
  [Vd] -> Mux3/2
  [Vq] -> Mux3/1
  Synchronous Machine pu Fundamental/1 -> Bus Selector3/1
  Mux3/1 -> Positive Sequence Voltage2/1
  wref6/1 -> ST1A Excitation System/1
  Positive Sequence Voltage2/1 -> V/1
  [w] -> f/1
  Bus Selector3/9 -> [dTheta]  "<Rotor angle deviation  d_theta (rad)>"
  Mux1/1 -> Positive Sequence Voltage1/1
  [Vq] -> Mux1/2
  [Vd] -> Mux1/1
  Govenor/1(throttle) -> Reheat steam turbine dynamics/1
  [w] -> Govenor/2(speed)
  Reheat steam turbine dynamics/1 -> Synchronous Machine pu Fundamental/1  "Pm"
  wref7/1 -> Govenor/1(speed_ref)
  [Q] -> Q/1
  Pset/1 -> Govenor/3(P_set)
  [Q] -> Scope/2
  [Ifd] -> ST1A Excitation System/3
  Positive Sequence Voltage1/1 -> ST1A Excitation System/2
  connections:
  Synchronous Machine pu Fundamental/RConn2 -- B/RConn1
  C/RConn1 -- Synchronous Machine pu Fundamental/RConn3
  Synchronous Machine pu Fundamental/RConn1 -- A/RConn1

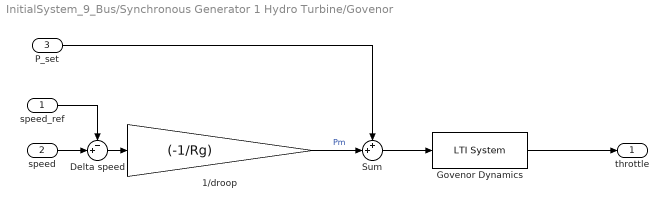
== system InitialSystem_9_Bus/Synchronous Generator 1 Hydro Turbine/Govenor ==
  speed_ref : Inport
  speed : Inport  Port=2
  P_set : Inport  Port=3
  1/droop : Gain  Gain=(-1/Rg)
  Delta speed : Sum  Inputs=-+|
  Govenor Dynamics : cstblocks/LTI System  sys=ss(HGov_dyn)  IC=[1 1.0617]
  Sum : Sum  Inputs=++|
  throttle : Outport  VectorParamsAs1DForOutWhenUnconnected=off
  wires:
  speed/1 -> Delta speed/2
  speed_ref/1 -> Delta speed/1
  Govenor Dynamics/1 -> throttle/1
  Delta speed/1 -> 1/droop/1
  Sum/1 -> Govenor Dynamics/1
  1/droop/1 -> Sum/2  "Pm"
  P_set/1 -> Sum/1

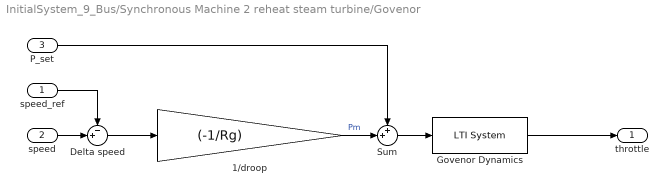
== system InitialSystem_9_Bus/Synchronous Machine 2 reheat steam turbine/Govenor ==
  speed_ref : Inport
  speed : Inport  Port=2
  P_set : Inport  Port=3
  1/droop : Gain  Gain=(-1/Rg)
  Delta speed : Sum  Inputs=-+|
  Govenor Dynamics : cstblocks/LTI System  sys=ss(SGov_dyn)  IC=[p_set_bus2/2.5]
  Sum : Sum  Inputs=++|
  throttle : Outport  VectorParamsAs1DForOutWhenUnconnected=off
  wires:
  speed/1 -> Delta speed/2
  speed_ref/1 -> Delta speed/1
  Govenor Dynamics/1 -> throttle/1
  Delta speed/1 -> 1/droop/1
  1/droop/1 -> Sum/2  "Pm"
  Sum/1 -> Govenor Dynamics/1
  P_set/1 -> Sum/1

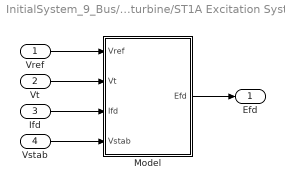
== system InitialSystem_9_Bus/Synchronous Machine 2 reheat steam turbine/ST1A Excitation System ==
  Vref : Inport
  Vt : Inport  Port=2
  Ifd : Inport  Port=3
  Vstab : Inport  Port=4
  Model : Subsystem  AncestorBlock=spsST1AModel/Continuous  mask(Excitation System){}
  Efd : Outport  VectorParamsAs1DForOutWhenUnconnected=off
  wires:
  Vstab/1 -> Model/4(Vstab)
  Ifd/1 -> Model/3(Ifd)
  Vref/1 -> Model/1(Vref)
  Vt/1 -> Model/2(Vt)
  Model/1(Efd) -> Efd/1

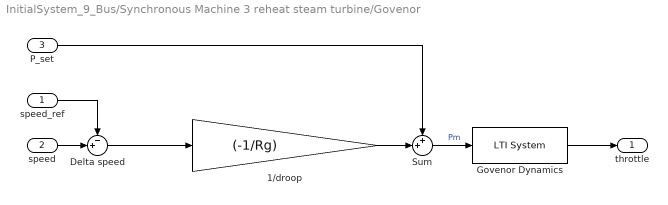
== system InitialSystem_9_Bus/Synchronous Machine 3 reheat steam turbine/Govenor ==
  speed_ref : Inport
  speed : Inport  Port=2
  P_set : Inport  Port=3
  1/droop : Gain  Gain=(-1/Rg)
  Delta speed : Sum  Inputs=-+|
  Govenor Dynamics : cstblocks/LTI System  sys=ss(SGov_dyn)  IC=[p_set_bus3/2.5]
  Sum : Sum  Inputs=++|
  throttle : Outport  VectorParamsAs1DForOutWhenUnconnected=off
  wires:
  speed/1 -> Delta speed/2
  speed_ref/1 -> Delta speed/1
  Govenor Dynamics/1 -> throttle/1
  Delta speed/1 -> 1/droop/1
  Sum/1 -> Govenor Dynamics/1  "Pm"
  1/droop/1 -> Sum/2
  P_set/1 -> Sum/1

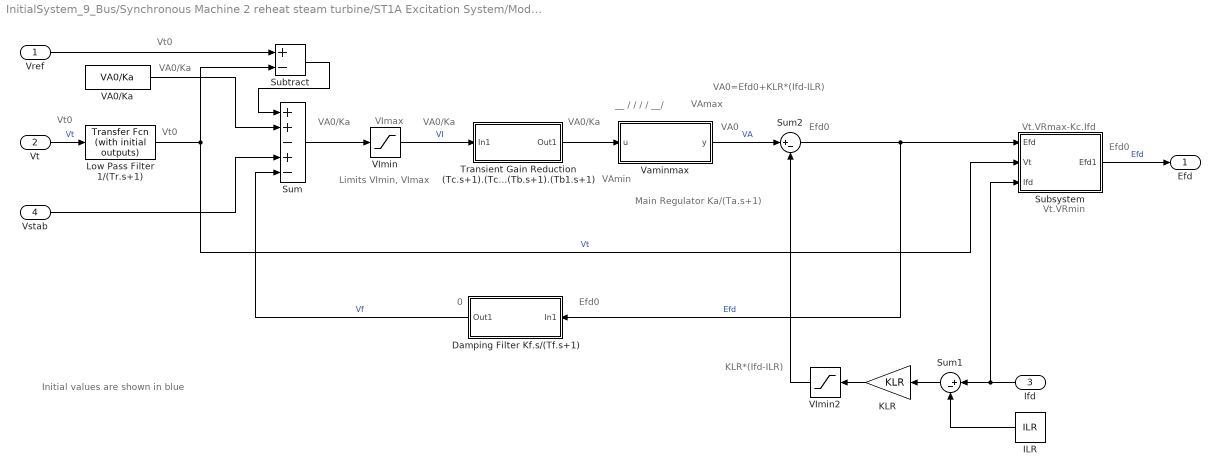
== system InitialSystem_9_Bus/Synchronous Machine 2 reheat steam turbine/ST1A Excitation System/Model ==
  note: Efd0
  note: Efd0
  note: VA0/Ka
  note: VA0/Ka
  note: Vt.VRmin
  note: VA0/Ka
  note: Efd0
  note: 0
  note: Vt0
  note: Vt.VRmax-Kc.Ifd
  note: Main Regulator
      | Ka/(Ta.s+1)
  note: VImax
  note: Initial values are shown in blue
  note: Vt0
  note: __
      |              /
      |           /
      |         /
      |       /
      | __/
  note: Limits VImin, VImax
  note: VAmax
  note: VAmin
  note: VA0/Ka
  note: KLR*(Ifd-ILR)
  note: VA0=Efd0+KLR*(Ifd-ILR)
  note: VA0
  note: Vt0
  Vref : Inport
  Vt : Inport  Port=2
  Ifd : Inport  Port=3
  Vstab : Inport  Port=4
  Damping Filter Kf.s/(Tf.s+1) : Subsystem  mask(Transfer Function with Initial Outputs){N=[Kf 0], D=[Tf 1], Y0=0, U0=Efd0}
      mask prompts: N "Numerator:"; D "Denominator:"; Y0 "Initial output:"; U0 "Initial input:"
      mask help: Vector expressions for numerator, and denominator. Coefficients are in descending powers of s.
      mask init:
      | [A,B,C,Dd]=tf2ss(N,D);
      | if (isempty(Y0));
      |     [m,n]=size(C);
      |     Y0=zeros(1,m); 
      | end; 
      | if (isempty(U0));
      |     [m,p]=size(B);
      |     U0=zeros(1,p);
      | end;
      | X0=getxo(A,B,C,Dd,U0,Y0,0);
      mask Help: Specify the initial output for the transfer function.  An optimization routine attempts to determine the appropriate initial states so that the specified initial output is achieved.  For more details, see the m-file getxo.m
      mask Display: dpoly(N,D,'s')
  ILR : Constant  Value=ILR
  KLR : Gain  Gain=KLR  SaturateOnIntegerOverflow=on  OutDataTypeStr=Inherit: Same as input  ParamDataTypeStr=Inherit: Same as input
  Low Pass Filter 1/(Tr.s+1) : simulink_extras/Additional Linear/Transfer Fcn (with initial outputs)  N=1  D=[Tr 1]  Y0=Vt0  U0=Vt0
  Subsystem : Subsystem
      mask Display: plot([0.15 0.85],[.5 .5],[.5 .5],[0.05 0.95],0.15+0.7*[0 .25 .75 1],0.05+0.9*[.25 .25 .75 .75]);
  Subtract : Sum  Inputs=+-
  Sum : Sum  Inputs=++-+-  InputSameDT=on  SaturateOnIntegerOverflow=on  OutDataTypeStr=Inherit: Same as first input
  Sum1 : Sum  Inputs=|+-  InputSameDT=on  SaturateOnIntegerOverflow=on  OutDataTypeStr=Inherit: Same as first input
  Sum2 : Sum  Inputs=|+-  InputSameDT=on  SaturateOnIntegerOverflow=on  OutDataTypeStr=Inherit: Same as first input
  Transient Gain Reduction (Tc.s+1).(Tc1.s+1) ----------------------- (Tb.s+1).(Tb1.s+1) : Subsystem  mask(Transfer Function with Initial Outputs){N=[Tc*Tc1 Tc+Tc1 1], D=[Tb*Tb1 Tb+Tb1 1], Y0=VA0/Ka, U0=VA0/Ka}
      mask prompts: N "Numerator:"; D "Denominator:"; Y0 "Initial output:"; U0 "Initial input:"
      mask help: Vector expressions for numerator, and denominator. Coefficients are in descending powers of s.
      mask init:
      | [A,B,C,Dd]=tf2ss(N,D);if (isempty(Y0));[m,n]=size(A);X0=zeros(1,m); end; if (isempty(U0));[m,p]=size(B);U0=zeros(1,p);end;
      |  if isempty(A),  X0=[]; else ,X0=getxo(A,B,C,Dd,U0,Y0,0); end
      mask Help: Specify the initial output for the transfer function.  An optimization routine attempts to determine the appropriate initial states so that the specified initial output is achieved.  For more details, see the m-file getxo.m
      mask Display: dpoly(N,D,'s')
  VA0/Ka : Constant  Value=VA0/Ka
  VImin : Saturate  UpperLimit=VImax  LowerLimit=VImin
  VImin2 : Saturate  UpperLimit=inf  LowerLimit=0
  Vaminmax : Subsystem  mask{Ka=Ka, Ta=Ta, VAminmax=[VAmin VAmax], X0=VA0}
      mask prompts: Ka "Voltage regulator gain Ka:"; Ta "Voltage regulator time constant Ta(s):"; VAminmax "Voltage regulator internal limits [VAmin(pu) VAmax(pu)]:"; X0 "Initial conditions:"
      mask init:
      | VAmin=VAminmax(1);VAmax=VAminmax(2);
      mask Display: dpoly([Ka],[Ta 1],'s')
  Efd : Outport
  wires:
  Ifd/1 -> Sum1/1, Subsystem/3(Ifd)
  Subsystem/1(Efd1) -> Efd/1  "Efd"
  Vt/1 -> Low Pass Filter 1/(Tr.s+1)/1  "Vt"
  Vaminmax/1(y) -> Sum2/1  "VA"
  Sum/1 -> VImin/1
  Sum1/1 -> KLR/1
  ILR/1 -> Sum1/2
  Sum2/1 -> Damping Filter Kf.s/(Tf.s+1)/1(In1), Subsystem/1(Efd)  "Efd"
  Transient Gain Reduction (Tc.s+1).(Tc1.s+1) ----------------------- (Tb.s+1).(Tb1.s+1)/1(Out1) -> Vaminmax/1(u)
  KLR/1 -> VImin2/1
  VA0/Ka/1 -> Sum/2
  Low Pass Filter 1/(Tr.s+1)/1 -> Subtract/2, Subsystem/2(Vt)  "Vt"
  VImin2/1 -> Sum2/2
  Damping Filter Kf.s/(Tf.s+1)/1(Out1) -> Sum/5  "Vf"
  VImin/1 -> Transient Gain Reduction (Tc.s+1).(Tc1.s+1) ----------------------- (Tb.s+1).(Tb1.s+1)/1(In1)  "VI"
  Vstab/1 -> Sum/4
  Vref/1 -> Subtract/1
  Subtract/1 -> Sum/1

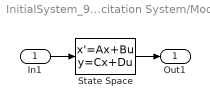
== system InitialSystem_9_Bus/Synchronous Machine 2 reheat steam turbine/ST1A Excitation System/Model/Damping Filter Kf.s//(Tf.s+1) ==
  In1 : Inport
  State Space : StateSpace  A=A  B=B  C=C  D=Dd  InitialCondition=X0
  Out1 : Outport  InitialOutput=0
  wires:
  In1/1 -> State Space/1
  State Space/1 -> Out1/1

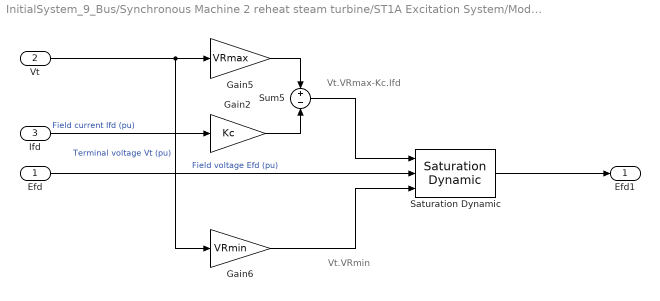
== system InitialSystem_9_Bus/Synchronous Machine 2 reheat steam turbine/ST1A Excitation System/Model/Subsystem ==
  note: Vt.VRmax-Kc.Ifd
  note: Vt.VRmin
  Efd : Inport
  Vt : Inport  Port=2
  Ifd : Inport  Port=3
  Gain2 : Gain  Gain=Kc  SaturateOnIntegerOverflow=on  OutDataTypeStr=Inherit: Same as input  ParamDataTypeStr=Inherit: Same as input
  Gain5 : Gain  Gain=VRmax  SaturateOnIntegerOverflow=on  OutDataTypeStr=Inherit: Same as input  ParamDataTypeStr=Inherit: Same as input
  Gain6 : Gain  Gain=VRmin  SaturateOnIntegerOverflow=on  OutDataTypeStr=Inherit: Same as input  ParamDataTypeStr=Inherit: Same as input
  Saturation Dynamic : simulink/Discontinuities/Saturation Dynamic  OutMin=[]  OutMax=[]  OutDataTypeStr=Inherit: Same as second input  OutDataType=fixdt(1, 16)  OutScaling=2^-10  DoSatur=off
  Sum5 : Sum  Inputs=+-  InputSameDT=on  SaturateOnIntegerOverflow=on  OutDataTypeStr=Inherit: Same as first input
  Efd1 : Outport
  wires:
  Gain2/1 -> Sum5/2
  Ifd/1 -> Gain2/1  "Field current Ifd (pu)"
  Efd/1 -> Saturation Dynamic/2  "Field voltage Efd (pu)"
  Gain6/1 -> Saturation Dynamic/3
  Saturation Dynamic/1 -> Efd1/1
  Gain5/1 -> Sum5/1
  Vt/1 -> Gain6/1, Gain5/1  "Terminal voltage Vt (pu)"
  Sum5/1 -> Saturation Dynamic/1

== system InitialSystem_9_Bus/Synchronous Machine 2 reheat steam turbine/ST1A Excitation System/Model/Transient Gain Reduction (Tc.s+1).(Tc1.s+1) ----------------------- (Tb.s+1).(Tb1.s+1) ==
  In1 : Inport
  State Space : StateSpace  A=A  B=B  C=C  D=Dd  InitialCondition=X0
  Out1 : Outport  InitialOutput=0
  wires:
  In1/1 -> State Space/1
  State Space/1 -> Out1/1
